simulink model "can_decoder"  (R2023b)
settings: configuration reference "AMCBLDC_Configuration" (kept outside this file)
undefined symbols (not defined in the file): CAN_ID_AMC, CAN_VOLT_REF_GAIN, CAN_VOLT_REF_SHIFT
settings Model: DataDictionary=amcbldc.sldd  Creator=upattacini  LastModifiedBy=mfussi
settings ConfigSetRef: SourceName=AMCBLDC_Configuration

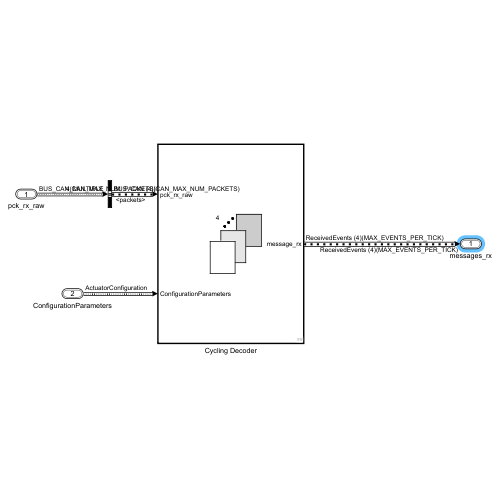
[thumbnail: Simulink's stored preview of the top-level diagram]
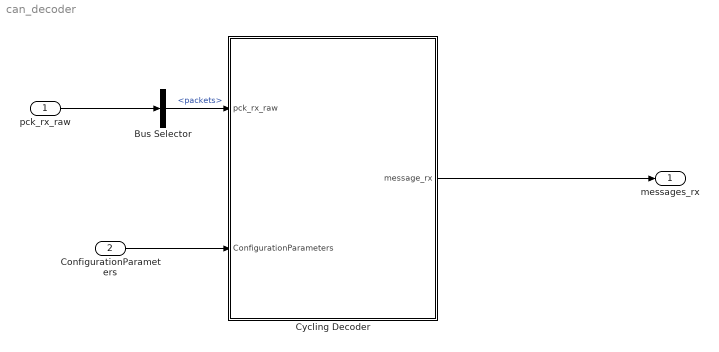
== system can_decoder ==
  pck_rx_raw : Inport  OutDataTypeStr=Bus: BUS_CAN_MULTIPLE  BusOutputAsStruct=on
  ConfigurationParameters : Inport  Port=2  OutDataTypeStr=Bus: ActuatorConfiguration  BusOutputAsStruct=on
  Bus Selector : BusSelector  OutputSignals=packets
  Cycling Decoder : Subsystem
  messages_rx : Outport  OutDataTypeStr=Bus: ReceivedEvents  BusOutputAsStruct=on
  wires:
  pck_rx_raw/1 -> Bus Selector/1
  Bus Selector/1 -> Cycling Decoder/1(pck_rx_raw)  "<packets>"
  ConfigurationParameters/1 -> Cycling Decoder/2(ConfigurationParameters)
  Cycling Decoder/1(message_rx) -> messages_rx/1

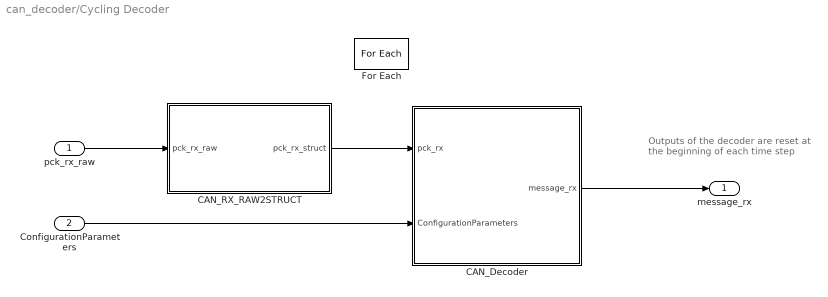
== system can_decoder/Cycling Decoder ==
  note: Outputs of the decoder are reset at
      | the beginning of each time step
  pck_rx_raw : Inport  Partition=on  PartitionDimension=1  PartitionWidth=1  PartitionOffset=0
  ConfigurationParameters : Inport  Port=2
  CAN_Decoder : Subsystem  TreatAsAtomicUnit=on
  CAN_RX_RAW2STRUCT : Subsystem  TreatAsAtomicUnit=on
  For Each : ForEach  DisableCoverage=on  SpecifiedNumIters=MAX_EVENTS_PER_TICK
  message_rx : Outport  OutDataTypeStr=Bus: ReceivedEvents  ConcatenationDimension=1
  wires:
  CAN_RX_RAW2STRUCT/1(pck_rx_struct) -> CAN_Decoder/1(pck_rx)
  pck_rx_raw/1 -> CAN_RX_RAW2STRUCT/1(pck_rx_raw)
  ConfigurationParameters/1 -> CAN_Decoder/2(ConfigurationParameters)
  CAN_Decoder/1(message_rx) -> message_rx/1

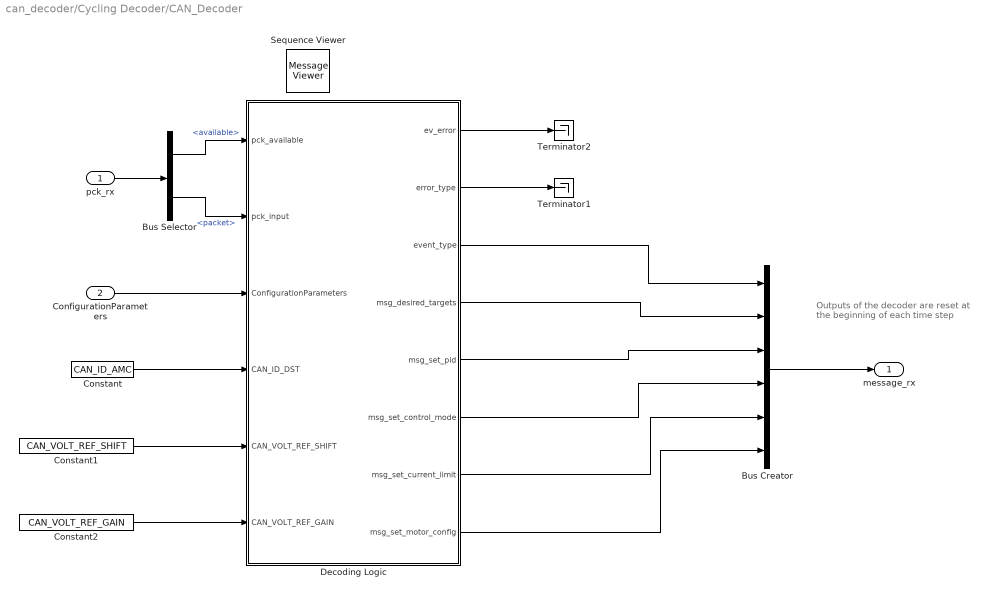
== system can_decoder/Cycling Decoder/CAN_Decoder ==
  note: Outputs of the decoder are reset at
      | the beginning of each time step
  pck_rx : Inport  OutDataTypeStr=Bus: BUS_CAN_RX
  ConfigurationParameters : Inport  Port=2  OutDataTypeStr=Bus: ActuatorConfiguration
  Bus Creator : BusCreator  Inputs=6  OutDataTypeStr=Bus: ReceivedEvents  NonVirtualBus=on
      settings: InheritFromInputs=off
  Bus Selector : BusSelector  OutputSignals=available,packet
  Constant : Constant  Value=CAN_ID_AMC  OutDataTypeStr=uint8
  Constant1 : Constant  Value=CAN_VOLT_REF_SHIFT  OutDataTypeStr=uint8
  Constant2 : Constant  Value=CAN_VOLT_REF_GAIN  OutDataTypeStr=single
  Decoding Logic : Stateflow chart  TreatAsAtomicUnit=on
      settings: PortSchema="{\"entries\":[{\"content\":{\"sides\":[{\"content\":{\"connectorIds\":[\"In1\",\"In2\",\"In3\",\"In4\",\"In5\",\"In6\"]},\"type\":\"ConnectorPlacement.EquallySpacedRectSide\",\"uuid\":\"bb5ffdcb-390f-4d7b-9f99-b75bae8a05ad\"},{\"content\":{\"connectorIds\":[\"Out8\",\"Out6\",\"Out7\",\"Out3\",\"Out4\",\"Out1\",\"Out2\",\"Out5\"],\"side\":\"RIGHT\"},\"type\":\"ConnectorPlacement.EquallySpacedRectSide\",\"uuid\":\"3ba90815-a3e4-4cd4-b64a-5c95e1f5d631\"},{\"content\":{\"side\":\"TOP\"},\"type\":\"ConnectorPlacement.EquallySpacedRectSide\",\"uuid\":\"c9c9b262-1031-4ca9-8b93-619604387376\"}]},\"type\":\"ConnectorPlacement.EquallySpacedConnector\",\"uuid\":\"025015ea-955c-40a8-a93e-b34368e10f0a\"}],\"packageUris\":[\"http://schema.mathworks.com/mf0/Connector/R2020b\"],\"version\":\"1.0\"}"
  Sequence Viewer : MessageViewer
  Terminator1 : Terminator
  Terminator2 : Terminator
  message_rx : Outport  OutDataTypeStr=Bus: ReceivedEvents
  wires:
  Constant/1 -> Decoding Logic/4(CAN_ID_DST)
  pck_rx/1 -> Bus Selector/1
  Bus Selector/1 -> Decoding Logic/1(pck_available)  "<available>"
  Bus Selector/2 -> Decoding Logic/2(pck_input)  "<packet>"
  ConfigurationParameters/1 -> Decoding Logic/3(ConfigurationParameters)
  Constant1/1 -> Decoding Logic/5(CAN_VOLT_REF_SHIFT)
  Constant2/1 -> Decoding Logic/6(CAN_VOLT_REF_GAIN)
  Decoding Logic/8(ev_error) -> Terminator2/1
  Decoding Logic/6(error_type) -> Terminator1/1
  Bus Creator/1 -> message_rx/1
  Decoding Logic/7(event_type) -> Bus Creator/1
  Decoding Logic/3(msg_desired_targets) -> Bus Creator/2
  Decoding Logic/4(msg_set_pid) -> Bus Creator/3
  Decoding Logic/1(msg_set_control_mode) -> Bus Creator/4
  Decoding Logic/2(msg_set_current_limit) -> Bus Creator/5
  Decoding Logic/5(msg_set_motor_config) -> Bus Creator/6

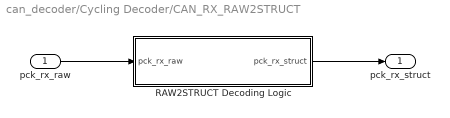
== system can_decoder/Cycling Decoder/CAN_RX_RAW2STRUCT ==
  pck_rx_raw : Inport  OutDataTypeStr=Bus: BUS_CAN
  RAW2STRUCT Decoding Logic : MATLAB Function  TreatAsAtomicUnit=on
  pck_rx_struct : Outport
  wires:
  pck_rx_raw/1 -> RAW2STRUCT Decoding Logic/1(pck_rx_raw)
  RAW2STRUCT Decoding Logic/1(pck_rx_struct) -> pck_rx_struct/1

== matlab function can_decoder/Cycling Decoder/CAN_RX_RAW2STRUCT/RAW2STRUCT Decoding Logic ==
  data: pck_rx_raw input Bus: BUS_CAN; pck_rx_struct output Bus: BUS_CAN_RX
function pck_rx_struct = raw2struct(pck_rx_raw)

pck_rx_struct.available = pck_rx_raw.available;

% ID
pck_rx_struct.packet.ID.CLS = CANClassTypes(bitshift(bitand(pck_rx_raw.packet.ID, 0x0700), -8));
pck_rx_struct.packet.ID.SRC = uint8(bitshift(bitand(pck_rx_raw.packet.ID, 0x0f0), -4));
pck_rx_struct.packet.ID.DST_TYP = uint8(bitand(pck_rx_raw.packet.ID, 0x00f));

% PAYLOAD
pck_rx_struct.packet.PAYLOAD.LEN = max([0, min([8, pck_rx_raw.length])]);
pck_rx_struct.packet.PAYLOAD.CMD.M = (bitand(pck_rx_raw.packet.PAYLOAD(1), 0x80) ~= 0);
pck_rx_struct.packet.PAYLOAD.CMD.OPC = bitand(pck_rx_raw.packet.PAYLOAD(1), 0x7f);

% We get both the polling and the streaming packtes covered
pck_rx_struct.packet.PAYLOAD.ARG = pck_rx_raw.packet.PAYLOAD;

== stateflow chart can_decoder/Cycling Decoder/CAN_Decoder/Decoding Logic ==
  settings: initializeOutput=1  description=This state chart is responsible for decoding incoming CAN packets.
  state SET_CONTROL_MODE [parallel]
    settings: executionOrder=1
    state Home
    (default) -> SET_CONTROL_MODE.Home
    (junction 24) -> SET_CONTROL_MODE.Home [order 1] : [is_controlmode_recognized(mc_mode)]
        | {% msg_set_control_mode.motor = pck_input.PAYLOAD.CMD.M;
        | msg_set_control_mode = convertMode(mc_mode);
        | cmd_processed++;
        | event_type = EventTypes.SetControlMode;}
    (junction 24) -> SET_CONTROL_MODE.Home [order 2] : /send(ev_error_mode_unrecognized, ERROR_HANDLING)
    (junction 22) -> SET_CONTROL_MODE.Home [order 2] : /send(ev_error_pck_malformed, ERROR_HANDLING)
    (junction 127) -> SET_CONTROL_MODE.Home [order 2]
    (junction 18) -> SET_CONTROL_MODE.Home [order 2] : /send(ev_error_pck_malformed, ERROR_HANDLING)
    SET_CONTROL_MODE.Home -> (junction 122) : [pck_available && (pck_input.ID.CLS == CANClassTypes.Motor_Control_Command)]
    (junction 122) -> SET_CONTROL_MODE.Home [order 2] : /send(ev_error_pck_not4us, ERROR_HANDLING)
    (junction 122) -> (junction 18) [order 1] : [pck_input.ID.DST_TYP == CAN_ID_DST]
    (junction 18) -> (junction 127) [order 1] : [pck_input.PAYLOAD.LEN >= 1]
    (junction 127) -> (junction 22) [order 1] : [pck_input.PAYLOAD.CMD.OPC == MCOPC.Set_Control_Mode]
    (junction 22) -> (junction 24) [order 1] : [pck_input.PAYLOAD.LEN >= 2]
        | {mc_mode = pck_input.PAYLOAD.ARG[1];}
  state DESIRED_TARGETS [parallel]
    settings: executionOrder=2
    state Home
    (default) -> DESIRED_TARGETS.Home
    (junction 144) -> DESIRED_TARGETS.Home [order 1] : [(pck_input.PAYLOAD.LEN == 8) && (CAN_ID_DST <= 4)]
        | {idx = 2*(CAN_ID_DST-1);
        | tmp_merged = merge_2bytes_signed(pck_input.PAYLOAD.ARG[idx], pck_input.PAYLOAD.ARG[idx+1]);
        | msg_desired_targets.current = single(0.001) * single(tmp_merged);
        | msg_desired_targets.voltage = single(tmp_merged >> (CAN_VOLT_REF_SHIFT - ConfigurationParameters.pids.currentPID.shift_factor)) / CAN_VOLT_REF_GAIN;
        | msg_desired_targets.velocity = single(1000) * single(tmp_merged) * CAN_ANGLE_ICUB2DEG;
        | cmd_processed++;
        | event_type = EventTypes.SetTarget;}
    (junction 144) -> DESIRED_TARGETS.Home [order 2] : /send(ev_error_pck_malformed, ERROR_HANDLING)
    DESIRED_TARGETS.Home -> (junction 144) : [pck_available && (pck_input.ID.CLS == CANClassTypes.Motor_Control_Streaming) && (MCStreaming(pck_input.ID.DST_TYP) == MCStreaming.Desired_Targets)]
  state SET_OPTIONS [parallel]
    settings: executionOrder=3
    note: velocity PID gains are supposed to be in mA/(deg/s)
        | whereas the current loop is in A
    state Home
    (junction 249) -> SET_OPTIONS.Home
    (junction 247) -> (junction 249) [order 2] : {msg_set_pid.P *= single(0.001);
        | msg_set_pid.I *= single(0.001);
        | msg_set_pid.D *= single(0.001);
        | msg_set_pid.type = ControlModes.Velocity;
        | event_type = EventTypes.SetPid;}
    (junction 247) -> (junction 249) [order 1] : [pck_input.PAYLOAD.CMD.OPC == MCOPC.Set_Current_PID]
        | {event_type = EventTypes.SetPid;}
    (default) -> SET_OPTIONS.Home
    (junction 135) -> SET_OPTIONS.Home [order 1] : [pck_input.PAYLOAD.LEN == 8]
        | {
        | % msg_set_current_limit.motor = pck_input.PAYLOAD.CMD.M;
        | msg_set_current_limit.nominal = single(0.001)*single(merge_2bytes_signed(pck_input.PAYLOAD.ARG[2], pck_input.PAYLOAD.ARG[3]));
        | msg_set_current_limit.peak = single(0.001)*single(merge_2bytes_unsigned(pck_input.PAYLOAD.ARG[4], pck_input.PAYLOAD.ARG[5]));
        | msg_set_current_limit.overload = single(0.001)*single(merge_2bytes_unsigned(pck_input.PAYLOAD.ARG[6], pck_input.PAYLOAD.ARG[7]));
        | cmd_processed++;
        | event_type = EventTypes.SetLimit;}
    (junction 203) -> SET_OPTIONS.Home : /send(ev_error_pck_malformed, ERROR_HANDLING)
    (junction 132) -> SET_OPTIONS.Home [order 3]
    (junction 58) -> SET_OPTIONS.Home [order 2] : /send(ev_error_pck_malformed, ERROR_HANDLING)
    SET_OPTIONS.Home -> (junction 124) : [pck_available && (pck_input.ID.CLS == CANClassTypes.Motor_Control_Command)]
    (junction 124) -> SET_OPTIONS.Home [order 2] : /send(ev_error_pck_not4us, ERROR_HANDLING)
    (junction 124) -> (junction 58) [order 1] : [pck_input.ID.DST_TYP == CAN_ID_DST]
    (junction 132) -> (junction 135) [order 1] : [pck_input.PAYLOAD.CMD.OPC == MCOPC.Set_Current_Limit]
    (junction 135) -> (junction 203) [order 2]
    (junction 58) -> (junction 132) [order 1] : [pck_input.PAYLOAD.LEN >= 1]
    (junction 132) -> (junction 200) [order 2] : [(pck_input.PAYLOAD.CMD.OPC == MCOPC.Set_Current_PID) || (pck_input.PAYLOAD.CMD.OPC == MCOPC.Set_Velocity_PID)]
    (junction 200) -> (junction 247) [order 1] : [pck_input.PAYLOAD.LEN == 8]
        | {
        | % msg_set_pid.motor = pck_input.PAYLOAD.CMD.M;
        | msg_set_pid.shift_factor = pck_input.PAYLOAD.ARG[7];
        | c = single(0x01 << (15 - msg_set_pid.shift_factor)) / single(32768);
        | msg_set_pid.P = c * single(merge_2bytes_signed(pck_input.PAYLOAD.ARG[1], pck_input.PAYLOAD.ARG[2]));
        | msg_set_pid.I = c * single(merge_2bytes_signed(pck_input.PAYLOAD.ARG[3], pck_input.PAYLOAD.ARG[4]));
        | msg_set_pid.D = c * single(merge_2bytes_signed(pck_input.PAYLOAD.ARG[5], pck_input.PAYLOAD.ARG[6]));
        | msg_set_pid.type = ControlModes.Current;
        | cmd_processed++;}
    (junction 200) -> (junction 203) [order 2]
  state SET_MOTOR_CONFIG [parallel]
    settings: executionOrder=4
    state Home
    (default) -> SET_MOTOR_CONFIG.Home
    (junction 261) -> SET_MOTOR_CONFIG.Home [order 1] : [pck_input.PAYLOAD.LEN == 8]
        | {
        | msg_set_motor_config.has_quadrature_encoder = boolean(pck_input.PAYLOAD.ARG[1] & 0x01);
        | msg_set_motor_config.has_hall_sens = boolean(pck_input.PAYLOAD.ARG[1] & 0x02);
        | msg_set_motor_config.has_torque_sens = boolean(pck_input.PAYLOAD.ARG[1] & 0x04);
        | msg_set_motor_config.use_index = boolean(pck_input.PAYLOAD.ARG[1] & 0x08);
        | msg_set_motor_config.has_speed_quadrature_encoder = boolean(pck_input.PAYLOAD.ARG[1] & 0x10);
        | msg_set_motor_config.enable_verbosity = boolean(pck_input.PAYLOAD.ARG[1] & 0x20);
        | msg_set_motor_config.rotor_encoder_resolution = merge_2bytes_signed(pck_input.PAYLOAD.ARG[2], pck_input.PAYLOAD.ARG[3]);
        | msg_set_motor_config.rotor_index_offset = merge_2bytes_signed(pck_input.PAYLOAD.ARG[4], pck_input.PAYLOAD.ARG[5]);
        | msg_set_motor_config.pole_pairs = pck_input.PAYLOAD.ARG[6] / 2;
        | msg_set_motor_config.encoder_tolerance = pck_input.PAYLOAD.ARG[7];
        | cmd_processed++;
        | event_type = EventTypes.SetMotorConfig;}
    (junction 263) -> SET_MOTOR_CONFIG.Home [order 2]
    (junction 262) -> SET_MOTOR_CONFIG.Home [order 2] : /send(ev_error_pck_malformed, ERROR_HANDLING)
    SET_MOTOR_CONFIG.Home -> (junction 260) : [pck_available && (pck_input.ID.CLS == CANClassTypes.Motor_Control_Command)]
    (junction 260) -> SET_MOTOR_CONFIG.Home [order 2] : /send(ev_error_pck_not4us, ERROR_HANDLING)
    (junction 261) -> SET_MOTOR_CONFIG.Home [order 2] : /send(ev_error_pck_malformed, ERROR_HANDLING)
    (junction 260) -> (junction 262) [order 1] : [pck_input.ID.DST_TYP == CAN_ID_DST]
    (junction 262) -> (junction 263) [order 1] : [pck_input.PAYLOAD.LEN >= 1]
    (junction 263) -> (junction 261) [order 1] : [pck_input.PAYLOAD.CMD.OPC == MCOPC.Set_Motor_Config]
  state ERROR_HANDLING [parallel]
    settings: executionOrder=5
    state Home
      entry:
      cmd_processed = 0;
      exit:
      ev_async = false;
    state Event_Error
      entry:
      ev_async = true;
    (default) -> ERROR_HANDLING.Home
    (junction 111) -> ERROR_HANDLING.Home [order 2] : {error_type = CANErrorTypes.No_Error;}
    (junction 111) -> ERROR_HANDLING.Home [order 1] : [cmd_processed > 1]
        | {error_type = CANErrorTypes.Packet_MultiFunctionsDetected;
        | send(ev_error);}
    ERROR_HANDLING.Home -> ERROR_HANDLING.Home [order 4] : [ev_async]
    (junction 109) -> ERROR_HANDLING.Home [order 1] : [pck_available && (cmd_processed == 0)]
        | {error_type = CANErrorTypes.Packet_Unrecognized;
        | send(ev_error);}
    Event_Error -> ERROR_HANDLING.Home
    ERROR_HANDLING.Home -> Event_Error [order 1] : ev_error_pck_not4us
        | {error_type = CANErrorTypes.Packet_Not4Us;
        | send(ev_error);}
    ERROR_HANDLING.Home -> Event_Error [order 2] : ev_error_pck_malformed
        | {error_type = CANErrorTypes.Packet_Malformed;
        | send(ev_error);}
    ERROR_HANDLING.Home -> Event_Error [order 3] : ev_error_mode_unrecognized
        | {error_type = CANErrorTypes.Mode_Unrecognized;
        | send(ev_error);}
    ERROR_HANDLING.Home -> (junction 109) [order 5]
    (junction 109) -> (junction 111) [order 2]
  data: MCMode function_input Enum: MCControlModes; mode function_output Enum: ControlModes; mc_mode local int32 size=1; idx local uint8; tmp_merged local int16; c local single; bl function_input uint16; bh function_input uint16; uw function_output uint16; bl function_input uint16; bh function_input uint16; sw function_output int16; mode function_input int32; ok function_output boolean; ev_async local boolean =false; pck_available input boolean; pck_input input Bus: BUS_CAN_PACKET_RX; ConfigurationParameters input Bus: ActuatorConfiguration; CAN_ID_DST input uint8; msg_set_control_mode output Enum: ControlModes; msg_set_current_limit output Bus: SupervisorInputLimits; msg_desired_targets output Bus: Targets; msg_set_pid output Bus: PID; msg_set_motor_config output Bus: MotorConfigurationExternal; error_type output Enum: CANErrorTypes size=1 =CANErrorTypes.No_Error; cmd_processed local uint16 size=1 =0; CAN_VOLT_REF_SHIFT input uint8; CAN_VOLT_REF_GAIN input single; CAN_ANGLE_ICUB2DEG parameter; event_type output Enum: EventTypes =EventTypes.None
  data mc_mode settings: description=Temporary variable.
  data CAN_ID_DST settings: description=The ID of the receiver.
  data msg_set_control_mode settings: description=Contains the data to set the required control mode.
  data msg_set_current_limit settings: description=Contains the data to set the required current limit.
  data msg_desired_targets settings: description=Contains the data to set the required current limit.
  data msg_set_pid settings: description=Contains the data to set the required current limit.
  data msg_set_motor_config settings: description=Contains the data to set the required current limit.
  events: ev_error_mode_unrecognized local FUNCTION_CALL_EVENT; ev_error output EITHER_EDGE_EVENT; ev_error_pck_malformed local FUNCTION_CALL_EVENT; ev_error_pck_not4us local FUNCTION_CALL_EVENT
  function mode = convertMode(MCMode):
    | function mode = convertMode(MCMode)
    | 
    |     if MCMode == MCControlModes.Idle
    |         mode = ControlModes.Idle;
    |     elseif MCMode == MCControlModes.Current
    |         mode = ControlModes.Current;
    |     elseif MCMode == MCControlModes.SpeedVoltage
    |         mode = ControlModes.Velocity;
    |     elseif MCMode == MCControlModes.OpenLoop
    |         mode = ControlModes.Voltage;
    |     else
    |         mode = ControlModes.Idle;
    |     end
    | 
    | end
  function uw = merge_2bytes_unsigned(bl, bh):
    | function uw = merge_2bytes_unsigned(bl, bh)
    | 
    | uw = bitor(bitshift(bh, 8), bl);
  function sw = merge_2bytes_signed(bl, bh):
    | function sw = merge_2bytes_signed(bl, bh)
    | 
    | uw = bitor(bitshift(bh, 8), bl);
    | sw = typecast(uw, 'int16');
  function ok = is_controlmode_recognized(mode):
    | function ok = is_controlmode_recognized(mode) 
    | 
    | ok = true;
    | if (mode ~= MCControlModes.Idle)         && ...
    |    (mode ~= MCControlModes.OpenLoop)     && ...
    |    (mode ~= MCControlModes.SpeedVoltage) && ...
    |    (mode ~= MCControlModes.Current)
    |     ok = false;
    | end
